simulink model "Energy_Storage_Project_2023a"  (R2023a)
settings: Solver=ode15s  StartTime=0.0  StopTime=1407  FixedStep=0.02  MaxStep=0.1  RelTol=1e-3
undefined symbols (not defined in the file or in its folder): C1, C2, par_balancing_type, R0, R1, R2, R_balance, SoC, V0, V1, V2, V3, V_ocv
libraries: fl_lib x44, nesl_utility x40, ee_lib x8
settings Model: NumberOfSteps=100  Creator=venka  LastModifiedBy=venka
settings RTWCC: GPUComputeCapability=5.0
settings ConfigComp: CovBoundaryAbsTol=1.0e-5

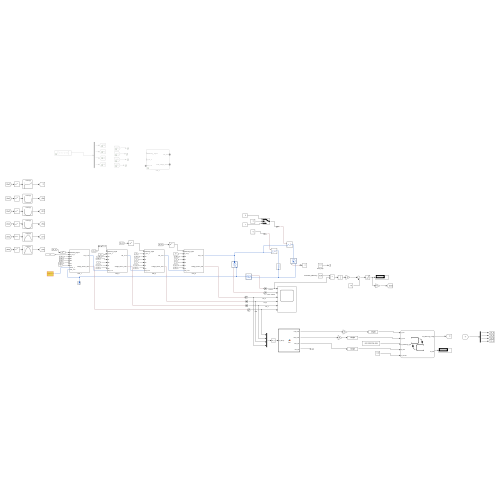
[thumbnail: Simulink's stored preview of the top-level diagram]
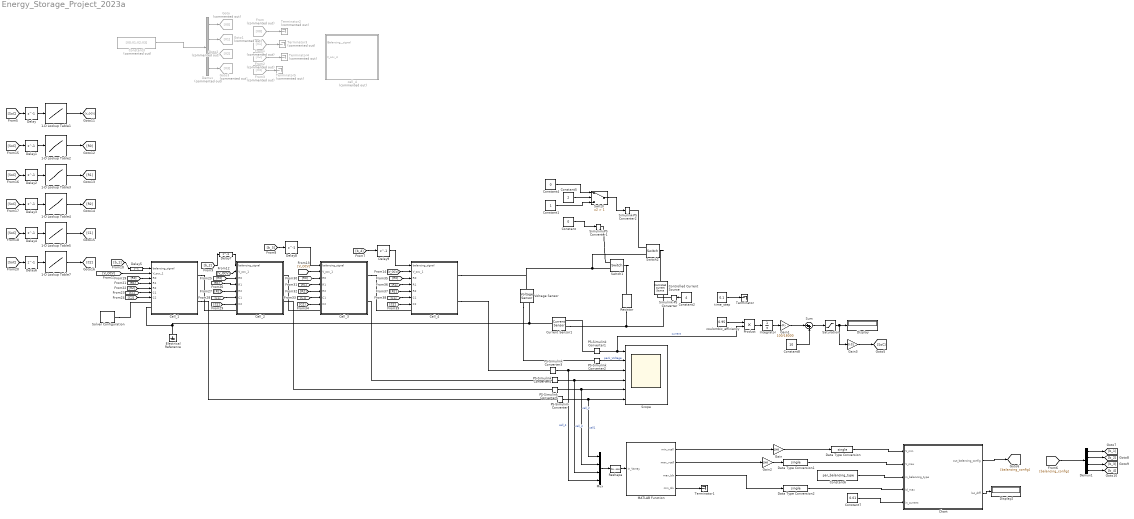
== system Energy_Storage_Project_2023a ==
  1-D Lookup Table1 : Lookup_n-D  NumberOfTableDimensions=1  BreakpointsForDimension1=SoC  Table=V_ocv  InternalRulePriority=Speed  RndMeth=Simplest
  1-D Lookup Table2 : Lookup_n-D  NumberOfTableDimensions=1  BreakpointsForDimension1=SoC  Table=R0  InternalRulePriority=Speed  RndMeth=Simplest
  1-D Lookup Table3 : Lookup_n-D  NumberOfTableDimensions=1  BreakpointsForDimension1=SoC  Table=R1  InternalRulePriority=Speed  RndMeth=Simplest
  1-D Lookup Table4 : Lookup_n-D  NumberOfTableDimensions=1  BreakpointsForDimension1=SoC  Table=R2  InternalRulePriority=Speed  RndMeth=Simplest
  1-D Lookup Table5 : Lookup_n-D  NumberOfTableDimensions=1  BreakpointsForDimension1=SoC  Table=C1  InternalRulePriority=Speed  RndMeth=Simplest
  1-D Lookup Table7 : Lookup_n-D  NumberOfTableDimensions=1  BreakpointsForDimension1=SoC  Table=C2  InternalRulePriority=Speed  RndMeth=Simplest
  Cell_1 : Subsystem
  Cell_2 : Subsystem
  Cell_3 : Subsystem
  Cell_4 : Subsystem
  Chart : Stateflow chart  TreatAsAtomicUnit=on
  Constant : Constant  Value=0
  Constant1 : Constant
  Constant2 : Constant  Value=4
  Constant3 : Constant  Commented=on  Value=[V0;V1;V2;V3]
  Constant4 : Constant  Value=0
  Constant5 : Constant  Value=2
  Constant6 : Constant  Value=par_balancing_type
  Constant7 : Constant  Value=0.01
  Constant8 : Constant  Value=10
  Controlled Current Source : fl_lib/Electrical/Electrical Sources/Controlled Current Source
  Current Sensor1 : fl_lib/Electrical/Electrical Sensors/Current Sensor
  Data Type Conversion : DataTypeConversion  OutDataTypeStr=single  SaturateOnIntegerOverflow=off  RndMeth=Floor
  Data Type Conversion1 : DataTypeConversion  OutDataTypeStr=single  SaturateOnIntegerOverflow=off  RndMeth=Floor
  Data Type Conversion2 : DataTypeConversion  OutDataTypeStr=single  SaturateOnIntegerOverflow=off  RndMeth=Floor
  Delay{,1..9} (10 alike) : Delay  DelayLength=1  InputProcessing=Columns as channels (frame based)
  Demux : Demux  Commented=on
  Demux1 : Demux
  Display : Display
  Display2 : Display
  Electrical Reference : fl_lib/Electrical/Electrical Elements/Electrical Reference
  From : From  Commented=on  GotoTag=V0
  From1 : From  Commented=on  GotoTag=V1
  From2 : From  Commented=on  GotoTag=V2
  From3 : From  Commented=on  GotoTag=V3
  Gain : Gain  Gain=1000
  Gain1 : Gain  Gain=100/18000
  Gain2 : Gain  Gain=1000
  Gain3 : Gain  Gain=0.01
  Goto : Goto  Commented=on  GotoTag=V0
  Goto1 : Goto  Commented=on  GotoTag=V1
  Goto2 : Goto  Commented=on  GotoTag=V2
  Goto3 : Goto  Commented=on  GotoTag=V3
  Integrator : Integrator
  MATLAB Function : MATLAB Function  TreatAsAtomicUnit=on
  Mux : Mux
  PS-Simulink Converter{,1..5} (6 alike) : nesl_utility/PS-Simulink Converter  PhysicalDomain=network_engine_domain  SubClassName=ps_output  LeftPortType=input  RightPortType=output  PseudoPeriodic=off  Frequencies=[]  VectorFormat=inherit  Unit=inherit  AffineConversion=off
  Product : Product
  Reshape : Reshape
  Resistor : fl_lib/Electrical/Electrical Elements/Resistor  R=0.33 Ohm  i_specify=off  i_priority=None  i=0 A  i_nominal_specify=off  i_nominal_value=1  i_nominal_unit=A  v_specify=off  v_priority=None  v=0 V  v_nominal_specify=off  v_nominal_value=1  v_nominal_unit=V
  Saturation : Saturate  UpperLimit=100  LowerLimit=0
  Scope : Scope  NumInputPorts=6
  Simulink-PS Converter : nesl_utility/Simulink-PS Converter  PhysicalDomain=network_engine_domain  SubClassName=ps_input  LeftPortType=input  RightPortType=output  PseudoPeriodic=off  Frequencies=[]  NoiseDistribution=none  NoiseParameters=[]  Unit=1  AffineConversion=off  FilteringAndDerivatives=provide  SimscapeFilterOrder=1  InputFilterTimeConstant=0.001  UdotUserProvided=0
  Simulink-PS Converter1 : nesl_utility/Simulink-PS Converter  PhysicalDomain=network_engine_domain  SubClassName=ps_input  LeftPortType=input  RightPortType=output  PseudoPeriodic=off  Frequencies=[]  NoiseDistribution=none  NoiseParameters=[]  Unit=1  AffineConversion=off  FilteringAndDerivatives=provide  SimscapeFilterOrder=1  InputFilterTimeConstant=0.001  UdotUserProvided=0
  Simulink-PS Converter2 : nesl_utility/Simulink-PS Converter  PhysicalDomain=network_engine_domain  SubClassName=ps_input  LeftPortType=input  RightPortType=output  PseudoPeriodic=off  Frequencies=[]  NoiseDistribution=none  NoiseParameters=[]  Unit=1  AffineConversion=off  FilteringAndDerivatives=provide  SimscapeFilterOrder=1  InputFilterTimeConstant=0.001  UdotUserProvided=0
  Solver Configuration : nesl_utility/Solver Configuration  PhysicalDomain=network_engine_domain  SubClassName=solver  LeftPortType=input  RightPortType=generic  Tones=[]  Harmonics=[]  SimulateNoise=off  Profile=off  UseLocalSampling=off  EnableSwitchedLinearOptims=on  FrequencyDomain=off  UseCCode=off  RelTol=0.001  AbsTol=0.001  MinStep=1e-09  ToWorkspace=off  RevertToSquareIcSolve=off  NumHomotopyIterations=100  PhasorMode=off  PhasorModeNumHarmonics=1  ConsistencySolver=NEWTON_XTOL_AFTER_FTOL  IndexReductionMethod=DerivativeReplacement  DoDC=off  ResidualTolerance=1e-09  ConsistencyTolSource=GLOBAL  ConsistencyAbsTol=0.001  ConsistencyRelTol=0.001  ConsistencyTolFactor=0.001  UseLocalSolver=off  LocalSolverChoice=NE_BACKWARD_EULER_ADVANCER  ResolveIndetEquations=on  FunctionEvalNumThread=1  LocalSolverSampleTime=0.001  DoFixedCost=off  MaxNonlinIter=3  MaxModeIter=2  ComputeImpulses=off  ImpulseIterations=2  LinearAlgebra=auto  LinearAlgebraNumThread=0  EquationFormulation=NE_TIME_EF  DelaysMemoryBudget=1024  AutomaticFiltering=on  FilteringTimeConstant=0.001  PartitionStorageMethod=AS_NEEDED  PartitionMemoryBudget=1024  PartitionMethod=ROBUST  MultibodyUseLocalSolver=off  MultibodyLocalSolverChoice=ODE1  MultibodyLocalSolverSampleTime=0.001
  Sum : Sum  Inputs=|++
  Switch : Switch  Criteria=u2 > Threshold  Threshold=1  SaturateOnIntegerOverflow=off  InputSameDT=off
  Switch1 : fl_lib/Electrical/Electrical Elements/Switch  R_closed=0.01 Ohm  G_open=1e-8 1/Ohm  Threshold=0.5  i_specify=off  i_priority=None  i=0 A  i_nominal_specify=off  i_nominal_value=1  i_nominal_unit=A  v_specify=off  v_priority=None  v=0 V  v_nominal_specify=off  v_nominal_value=1  v_nominal_unit=V
  Switch2 : fl_lib/Electrical/Electrical Elements/Switch  R_closed=0.01 Ohm  G_open=1e-8 1/Ohm  Threshold=0.5  i_specify=off  i_priority=None  i=0 A  i_nominal_specify=off  i_nominal_value=1  i_nominal_unit=A  v_specify=off  v_priority=None  v=0 V  v_nominal_specify=off  v_nominal_value=1  v_nominal_unit=V
  Terminator : Terminator
  Terminator1 : Terminator
  Terminator{2..5} (4 alike) : Terminator  Commented=on
  Voltage Sensor : fl_lib/Electrical/Electrical Sensors/Voltage Sensor
  cell_4 : Subsystem  Commented=on
  coulombic_efficiency : Constant  Value=0.95
  time_step : Constant  Value=0.1
  wires:
  PS-Simulink Converter/1 -> Scope/6, Mux/1  "cell1"
  PS-Simulink Converter1/1 -> Product/2, Scope/1  "current"
  PS-Simulink Converter2/1 -> Scope/2  "pack_Voltage"
  PS-Simulink Converter3/1 -> Mux/4, Scope/3  "cell_4"
  PS-Simulink Converter4/1 -> Mux/3, Scope/4  "cell_3"
  PS-Simulink Converter5/1 -> Scope/5, Mux/2  "cell_2"
  Constant2/1 -> Simulink-PS Converter/1
  Constant/1 -> Simulink-PS Converter1/1
  Constant3/1 -> Demux/1
  Demux/1 -> Goto/1
  Demux/2 -> Goto1/1
  Demux/3 -> Goto2/1
  Demux/4 -> Goto3/1
  time_step/1 -> Terminator/1
  coulombic_efficiency/1 -> Product/1
  Integrator/1 -> Gain1/1
  Product/1 -> Integrator/1
  Sum/1 -> Saturation/1
  Gain1/1 -> Sum/1
  Saturation/1 -> Gain3/1, Display/1
  Constant1/1 -> Switch/3
  Switch/1 -> Simulink-PS Converter2/1
  Constant4/1 -> Switch/1
  MATLAB Function/1(min_vcell) -> Gain/1
  MATLAB Function/2(max_vcell) -> Gain2/1
  Constant6/1 -> Chart/3(in_balancing_type)
  Data Type Conversion/1 -> Chart/1(V_min)
  Data Type Conversion1/1 -> Chart/2(V_max)
  MATLAB Function/3(max_Idx) -> Data Type Conversion2/1
  Data Type Conversion2/1 -> Chart/4(Id_max)
  [balancing_config] -> Demux1/1
  Demux1/1 -> [b_1]
  Demux1/2 -> [b_2]
  Demux1/3 -> [b_3]
  Demux1/4 -> [b_4]
  [b_3] -> Delay8/1
  Chart/1(out_balancing_config) -> [balancing_config]
  Constant5/1 -> Switch/2
  MATLAB Function/4(min_Idx) -> Terminator1/1
  Constant7/1 -> Chart/5(in_current)
  Gain/1 -> Data Type Conversion/1
  Gain2/1 -> Data Type Conversion1/1
  Chart/2(loc_diff) -> Display2/1
  From/1 -> Terminator2/1
  From1/1 -> Terminator3/1
  From2/1 -> Terminator4/1
  From3/1 -> Terminator5/1
  [SoC] -> Delay/1
  Delay/1 -> 1-D Lookup Table1/1
  1-D Lookup Table1/1 -> [V_OCV]
  [V_OCV] -> Cell_1/2(V_ocv_1)
  [V_OCV] -> Cell_2/2(V_ocv_1)
  [V_OCV] -> Cell_3/2(V_ocv_1)
  Constant8/1 -> Sum/2
  1-D Lookup Table2/1 -> [R0]
  [SoC] -> Delay1/1
  Delay1/1 -> 1-D Lookup Table2/1
  1-D Lookup Table3/1 -> [R1]
  [SoC] -> Delay2/1
  Delay2/1 -> 1-D Lookup Table3/1
  1-D Lookup Table4/1 -> [R2]
  [SoC] -> Delay3/1
  Delay3/1 -> 1-D Lookup Table4/1
  1-D Lookup Table5/1 -> [C1]
  [SoC] -> Delay4/1
  Delay4/1 -> 1-D Lookup Table5/1
  [b_4] -> Delay9/1
  [V_OCV] -> Cell_4/2(V_ocv_1)
  Delay6/1 -> 1-D Lookup Table7/1
  1-D Lookup Table7/1 -> [C2]
  [SoC] -> Delay6/1
  [R0] -> Cell_1/3(R0)
  [R1] -> Cell_1/4(R1)
  [R2] -> Cell_1/5(R2)
  [C1] -> Cell_1/6(C1)
  [C2] -> Cell_1/7(C2)
  [R1] -> Cell_2/4(R1)
  [R2] -> Cell_2/5(R2)
  [C2] -> Cell_2/7(C2)
  [C1] -> Cell_2/6(C1)
  [R0] -> Cell_2/3(R0)
  [R1] -> Cell_3/4(R1)
  [R2] -> Cell_3/5(R2)
  [C2] -> Cell_3/7(C2)
  [C1] -> Cell_3/6(C1)
  [R0] -> Cell_3/3(R0)
  [R1] -> Cell_4/4(R1)
  [R2] -> Cell_4/5(R2)
  [C2] -> Cell_4/7(C2)
  [C1] -> Cell_4/6(C1)
  [R0] -> Cell_4/3(R0)
  Mux/1 -> Reshape/1
  Reshape/1 -> MATLAB Function/1(in_Varray)
  [b_1] -> Delay5/1
  Delay5/1 -> Cell_1/1(balancing_signal)
  [b_2] -> Delay7/1
  Delay7/1 -> Cell_2/1(balancing_signal)
  Delay8/1 -> Cell_3/1(balancing_signal)
  Delay9/1 -> Cell_4/1(balancing_signal)
  Gain3/1 -> [SoC]
  connections:
  Switch2/RConn2 -- Cell_4/RConn1 -- Voltage Sensor/LConn1 -- Switch1/RConn2
  Switch1/LConn1 -- Resistor/LConn1
  Solver Configuration/RConn1 -- Cell_1/LConn1
  Cell_1/RConn1 -- Cell_2/LConn1
  Cell_3/LConn1 -- Cell_2/RConn1
  Electrical Reference/LConn1 -- Voltage Sensor/RConn2 -- Current Sensor1/LConn1 -- Cell_1/LConn2
  Cell_1/RConn2 -- PS-Simulink Converter/LConn1
  PS-Simulink Converter5/LConn1 -- Cell_2/RConn2
  PS-Simulink Converter4/LConn1 -- Cell_3/RConn2
  PS-Simulink Converter1/LConn1 -- Current Sensor1/RConn1
  Voltage Sensor/RConn1 -- PS-Simulink Converter2/LConn1
  Switch1/RConn1 -- Simulink-PS Converter1/RConn1
  Resistor/RConn1 -- Current Sensor1/RConn2 -- Controlled Current Source/RConn2
  Switch2/LConn1 -- Controlled Current Source/LConn1
  Switch2/RConn1 -- Simulink-PS Converter2/RConn1
  Simulink-PS Converter/RConn1 -- Controlled Current Source/RConn1
  Cell_3/RConn1 -- Cell_4/LConn1
  Cell_4/RConn2 -- PS-Simulink Converter3/LConn1

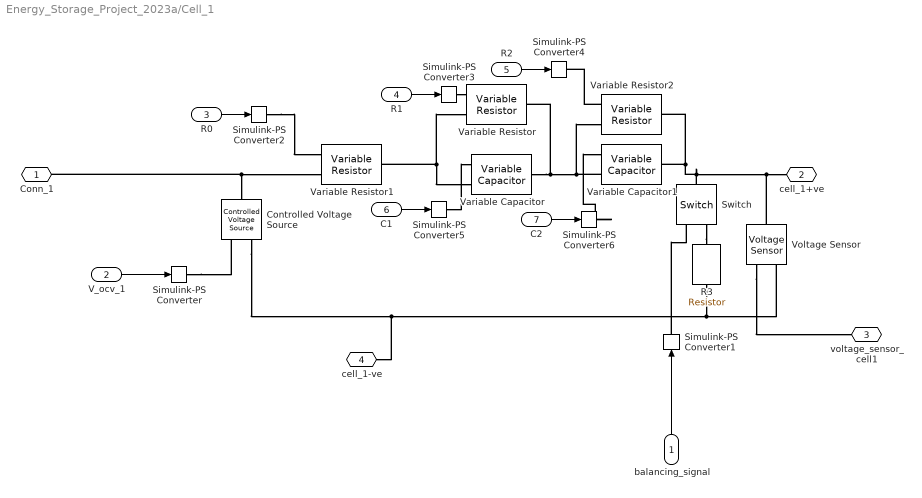
== system Energy_Storage_Project_2023a/Cell_1 ==
  balancing_signal : Inport
  V_ocv_1 : Inport  Port=2
  R0 : Inport  Port=3
  R1 : Inport  Port=4
  R2 : Inport  Port=5
  C1 : Inport  Port=6
  C2 : Inport  Port=7
  Controlled Voltage Source : fl_lib/Electrical/Electrical Sources/Controlled Voltage Source
  R3 : fl_lib/Electrical/Electrical Elements/Resistor  R=R_balance Ohm  i_specify=off  i_priority=None  i=0 A  i_nominal_specify=off  i_nominal_value=1  i_nominal_unit=A  v_specify=off  v_priority=None  v=0 V  v_nominal_specify=off  v_nominal_value=1  v_nominal_unit=V
  Simulink-PS Converter{,1..6} (7 alike) : nesl_utility/Simulink-PS Converter  PhysicalDomain=network_engine_domain  SubClassName=ps_input  LeftPortType=input  RightPortType=output  PseudoPeriodic=off  Frequencies=[]  NoiseDistribution=none  NoiseParameters=[]  Unit=1  AffineConversion=off  FilteringAndDerivatives=provide  SimscapeFilterOrder=1  InputFilterTimeConstant=0.001  UdotUserProvided=0
  Switch : fl_lib/Electrical/Electrical Elements/Switch  R_closed=0.01 Ohm  G_open=1e-8 1/Ohm  Threshold=0.5  i_specify=off  i_priority=None  i=0 A  i_nominal_specify=off  i_nominal_value=1  i_nominal_unit=A  v_specify=off  v_priority=None  v=0 V  v_nominal_specify=off  v_nominal_value=1  v_nominal_unit=V
  Variable Capacitor : ee_lib/Passive/Variable Capacitor  prm=2  Cmin=1e-9 F  r=1e-6 Ohm  v0=0 V  q0=0 C
      settings: InternalSimscapePortConfiguration="{\"Bottom\":[],\"Left\":[{\"id\":\"C\",\"label\":\"C\",\"type\":\"input\"},{\"id\":\"p\",\"label\":\"+\",\"type\":\"foundation.electrical.electrical\"}],\"Right\":[{\"id\":\"n\",\"label\":\"-\",\"type\":\"foundation.electrical.electrical\"}],\"Top\":[]}"
  Variable Capacitor1 : ee_lib/Passive/Variable Capacitor  prm=2  Cmin=1e-9 F  r=1e-6 Ohm  v0=0 V  q0=0 C
      settings: InternalSimscapePortConfiguration="{\"Bottom\":[],\"Left\":[{\"id\":\"C\",\"label\":\"C\",\"type\":\"input\"},{\"id\":\"p\",\"label\":\"+\",\"type\":\"foundation.electrical.electrical\"}],\"Right\":[{\"id\":\"n\",\"label\":\"-\",\"type\":\"foundation.electrical.electrical\"}],\"Top\":[]}"
  Variable Resistor : fl_lib/Electrical/Electrical Elements/Variable Resistor  Rmin=0 Ohm  thermalEnable=false  thermal_mass=1 J/K  i_specify=off  i_priority=None  i=0 A  i_nominal_specify=off  i_nominal_value=1  i_nominal_unit=A  v_specify=off  v_priority=None  v=0 V  v_nominal_specify=off  v_nominal_value=1  v_nominal_unit=V  T_specify=off  T_priority=None  T=300 K  T_nominal_specify=off  T_nominal_value=1  T_nominal_unit=K
  Variable Resistor1 : fl_lib/Electrical/Electrical Elements/Variable Resistor  Rmin=0 Ohm  thermalEnable=false  thermal_mass=1 J/K  i_specify=off  i_priority=None  i=0 A  i_nominal_specify=off  i_nominal_value=1  i_nominal_unit=A  v_specify=off  v_priority=None  v=0 V  v_nominal_specify=off  v_nominal_value=1  v_nominal_unit=V  T_specify=off  T_priority=None  T=300 K  T_nominal_specify=off  T_nominal_value=1  T_nominal_unit=K
  Variable Resistor2 : fl_lib/Electrical/Electrical Elements/Variable Resistor  Rmin=0 Ohm  thermalEnable=false  thermal_mass=1 J/K  i_specify=off  i_priority=None  i=0 A  i_nominal_specify=off  i_nominal_value=1  i_nominal_unit=A  v_specify=off  v_priority=None  v=0 V  v_nominal_specify=off  v_nominal_value=1  v_nominal_unit=V  T_specify=off  T_priority=None  T=300 K  T_nominal_specify=off  T_nominal_value=1  T_nominal_unit=K
  Voltage Sensor : fl_lib/Electrical/Electrical Sensors/Voltage Sensor
  Conn_1 : PMIOPort  Side=Left
  cell_1+ve : PMIOPort  Port=2  Side=Right
  voltage_sensor_cell1 : PMIOPort  Port=3  Side=Right
  cell_1-ve : PMIOPort  Port=4  Side=Left
  wires:
  V_ocv_1/1 -> Simulink-PS Converter/1
  balancing_signal/1 -> Simulink-PS Converter1/1
  R0/1 -> Simulink-PS Converter2/1
  R1/1 -> Simulink-PS Converter3/1
  R2/1 -> Simulink-PS Converter4/1
  C1/1 -> Simulink-PS Converter5/1
  C2/1 -> Simulink-PS Converter6/1
  connections:
  Voltage Sensor/LConn1 -- Variable Capacitor1/RConn1 -- Variable Resistor2/RConn1 -- Switch/LConn1 -- cell_1+ve/RConn1
  Variable Resistor1/RConn1 -- Variable Resistor/LConn2 -- Variable Capacitor/LConn2
  Variable Capacitor/RConn1 -- Variable Resistor/RConn1 -- Variable Capacitor1/LConn2 -- Variable Resistor2/LConn2
  cell_1-ve/RConn1 -- Controlled Voltage Source/RConn2 -- R3/RConn1 -- Voltage Sensor/RConn2
  Voltage Sensor/RConn1 -- voltage_sensor_cell1/RConn1
  Conn_1/RConn1 -- Variable Resistor1/LConn2 -- Controlled Voltage Source/LConn1
  Simulink-PS Converter/RConn1 -- Controlled Voltage Source/RConn1
  Switch/RConn2 -- R3/LConn1
  Simulink-PS Converter1/RConn1 -- Switch/RConn1
  Simulink-PS Converter2/RConn1 -- Variable Resistor1/LConn1
  Simulink-PS Converter3/RConn1 -- Variable Resistor/LConn1
  Variable Resistor2/LConn1 -- Simulink-PS Converter4/RConn1
  Simulink-PS Converter5/RConn1 -- Variable Capacitor/LConn1
  Simulink-PS Converter6/RConn1 -- Variable Capacitor1/LConn1

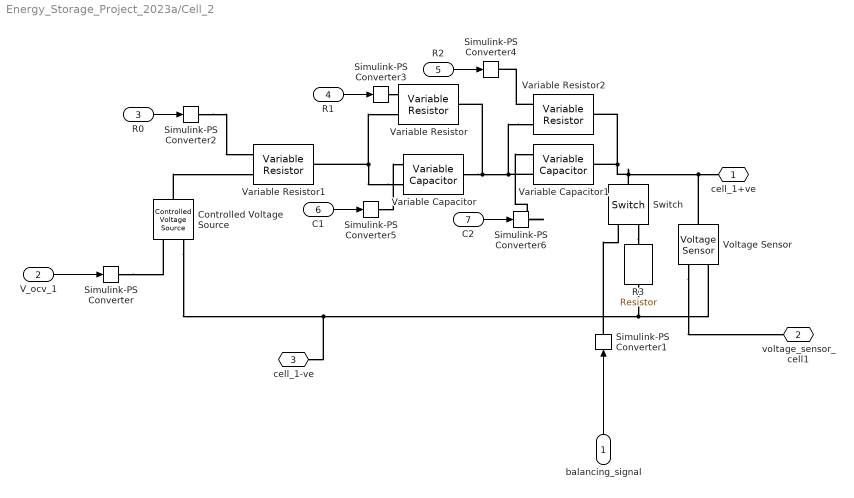
== system Energy_Storage_Project_2023a/Cell_2 ==
  balancing_signal : Inport
  V_ocv_1 : Inport  Port=2
  R0 : Inport  Port=3
  R1 : Inport  Port=4
  R2 : Inport  Port=5
  C1 : Inport  Port=6
  C2 : Inport  Port=7
  Controlled Voltage Source : fl_lib/Electrical/Electrical Sources/Controlled Voltage Source
  R3 : fl_lib/Electrical/Electrical Elements/Resistor  R=R_balance Ohm  i_specify=off  i_priority=None  i=0 A  i_nominal_specify=off  i_nominal_value=1  i_nominal_unit=A  v_specify=off  v_priority=None  v=0 V  v_nominal_specify=off  v_nominal_value=1  v_nominal_unit=V
  Simulink-PS Converter{,1..6} (7 alike) : nesl_utility/Simulink-PS Converter  PhysicalDomain=network_engine_domain  SubClassName=ps_input  LeftPortType=input  RightPortType=output  PseudoPeriodic=off  Frequencies=[]  NoiseDistribution=none  NoiseParameters=[]  Unit=1  AffineConversion=off  FilteringAndDerivatives=provide  SimscapeFilterOrder=1  InputFilterTimeConstant=0.001  UdotUserProvided=0
  Switch : fl_lib/Electrical/Electrical Elements/Switch  R_closed=0.01 Ohm  G_open=1e-8 1/Ohm  Threshold=0.5  i_specify=off  i_priority=None  i=0 A  i_nominal_specify=off  i_nominal_value=1  i_nominal_unit=A  v_specify=off  v_priority=None  v=0 V  v_nominal_specify=off  v_nominal_value=1  v_nominal_unit=V
  Variable Capacitor : ee_lib/Passive/Variable Capacitor  prm=2  Cmin=1e-9 F  r=1e-6 Ohm  v0=0 V  q0=0 C
      settings: InternalSimscapePortConfiguration="{\"Bottom\":[],\"Left\":[{\"id\":\"C\",\"label\":\"C\",\"type\":\"input\"},{\"id\":\"p\",\"label\":\"+\",\"type\":\"foundation.electrical.electrical\"}],\"Right\":[{\"id\":\"n\",\"label\":\"-\",\"type\":\"foundation.electrical.electrical\"}],\"Top\":[]}"
  Variable Capacitor1 : ee_lib/Passive/Variable Capacitor  prm=2  Cmin=1e-9 F  r=1e-6 Ohm  v0=0 V  q0=0 C
      settings: InternalSimscapePortConfiguration="{\"Bottom\":[],\"Left\":[{\"id\":\"C\",\"label\":\"C\",\"type\":\"input\"},{\"id\":\"p\",\"label\":\"+\",\"type\":\"foundation.electrical.electrical\"}],\"Right\":[{\"id\":\"n\",\"label\":\"-\",\"type\":\"foundation.electrical.electrical\"}],\"Top\":[]}"
  Variable Resistor : fl_lib/Electrical/Electrical Elements/Variable Resistor  Rmin=0 Ohm  thermalEnable=false  thermal_mass=1 J/K  i_specify=off  i_priority=None  i=0 A  i_nominal_specify=off  i_nominal_value=1  i_nominal_unit=A  v_specify=off  v_priority=None  v=0 V  v_nominal_specify=off  v_nominal_value=1  v_nominal_unit=V  T_specify=off  T_priority=None  T=300 K  T_nominal_specify=off  T_nominal_value=1  T_nominal_unit=K
  Variable Resistor1 : fl_lib/Electrical/Electrical Elements/Variable Resistor  Rmin=0 Ohm  thermalEnable=false  thermal_mass=1 J/K  i_specify=off  i_priority=None  i=0 A  i_nominal_specify=off  i_nominal_value=1  i_nominal_unit=A  v_specify=off  v_priority=None  v=0 V  v_nominal_specify=off  v_nominal_value=1  v_nominal_unit=V  T_specify=off  T_priority=None  T=300 K  T_nominal_specify=off  T_nominal_value=1  T_nominal_unit=K
  Variable Resistor2 : fl_lib/Electrical/Electrical Elements/Variable Resistor  Rmin=0 Ohm  thermalEnable=false  thermal_mass=1 J/K  i_specify=off  i_priority=None  i=0 A  i_nominal_specify=off  i_nominal_value=1  i_nominal_unit=A  v_specify=off  v_priority=None  v=0 V  v_nominal_specify=off  v_nominal_value=1  v_nominal_unit=V  T_specify=off  T_priority=None  T=300 K  T_nominal_specify=off  T_nominal_value=1  T_nominal_unit=K
  Voltage Sensor : fl_lib/Electrical/Electrical Sensors/Voltage Sensor
  cell_1+ve : PMIOPort  Side=Right
  voltage_sensor_cell1 : PMIOPort  Port=2  Side=Right
  cell_1-ve : PMIOPort  Port=3  Side=Left
  wires:
  V_ocv_1/1 -> Simulink-PS Converter/1
  balancing_signal/1 -> Simulink-PS Converter1/1
  R0/1 -> Simulink-PS Converter2/1
  R1/1 -> Simulink-PS Converter3/1
  R2/1 -> Simulink-PS Converter4/1
  C1/1 -> Simulink-PS Converter5/1
  C2/1 -> Simulink-PS Converter6/1
  connections:
  Voltage Sensor/LConn1 -- cell_1+ve/RConn1 -- Switch/LConn1 -- Variable Resistor2/RConn1 -- Variable Capacitor1/RConn1
  Variable Capacitor/LConn2 -- Variable Resistor1/RConn1 -- Variable Resistor/LConn2
  Variable Resistor2/LConn2 -- Variable Capacitor/RConn1 -- Variable Resistor/RConn1 -- Variable Capacitor1/LConn2
  cell_1-ve/RConn1 -- Controlled Voltage Source/RConn2 -- R3/RConn1 -- Voltage Sensor/RConn2
  Voltage Sensor/RConn1 -- voltage_sensor_cell1/RConn1
  Controlled Voltage Source/LConn1 -- Variable Resistor1/LConn2
  Simulink-PS Converter/RConn1 -- Controlled Voltage Source/RConn1
  Switch/RConn2 -- R3/LConn1
  Simulink-PS Converter1/RConn1 -- Switch/RConn1
  Simulink-PS Converter2/RConn1 -- Variable Resistor1/LConn1
  Simulink-PS Converter3/RConn1 -- Variable Resistor/LConn1
  Variable Resistor2/LConn1 -- Simulink-PS Converter4/RConn1
  Simulink-PS Converter5/RConn1 -- Variable Capacitor/LConn1
  Simulink-PS Converter6/RConn1 -- Variable Capacitor1/LConn1

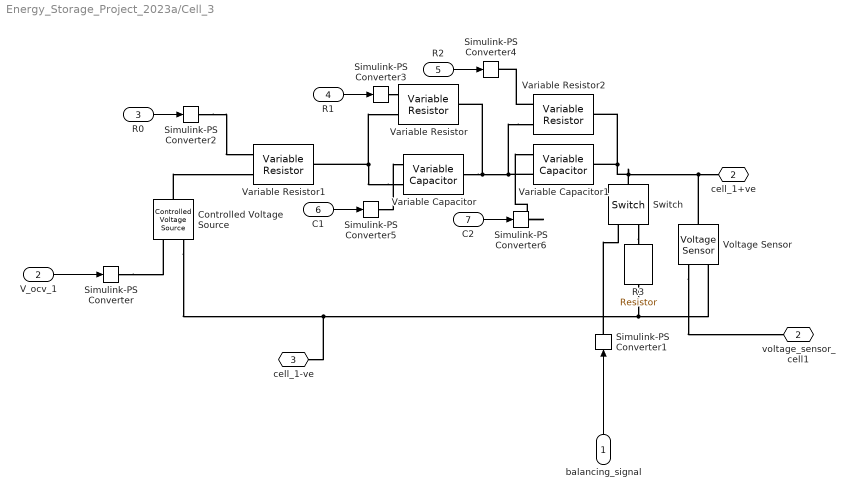
== system Energy_Storage_Project_2023a/Cell_3 ==
  balancing_signal : Inport
  V_ocv_1 : Inport  Port=2
  R0 : Inport  Port=3
  R1 : Inport  Port=4
  R2 : Inport  Port=5
  C1 : Inport  Port=6
  C2 : Inport  Port=7
  Controlled Voltage Source : fl_lib/Electrical/Electrical Sources/Controlled Voltage Source
  R3 : fl_lib/Electrical/Electrical Elements/Resistor  R=R_balance Ohm  i_specify=off  i_priority=None  i=0 A  i_nominal_specify=off  i_nominal_value=1  i_nominal_unit=A  v_specify=off  v_priority=None  v=0 V  v_nominal_specify=off  v_nominal_value=1  v_nominal_unit=V
  Simulink-PS Converter{,1..6} (7 alike) : nesl_utility/Simulink-PS Converter  PhysicalDomain=network_engine_domain  SubClassName=ps_input  LeftPortType=input  RightPortType=output  PseudoPeriodic=off  Frequencies=[]  NoiseDistribution=none  NoiseParameters=[]  Unit=1  AffineConversion=off  FilteringAndDerivatives=provide  SimscapeFilterOrder=1  InputFilterTimeConstant=0.001  UdotUserProvided=0
  Switch : fl_lib/Electrical/Electrical Elements/Switch  R_closed=0.01 Ohm  G_open=1e-8 1/Ohm  Threshold=0.5  i_specify=off  i_priority=None  i=0 A  i_nominal_specify=off  i_nominal_value=1  i_nominal_unit=A  v_specify=off  v_priority=None  v=0 V  v_nominal_specify=off  v_nominal_value=1  v_nominal_unit=V
  Variable Capacitor : ee_lib/Passive/Variable Capacitor  prm=2  Cmin=1e-9 F  r=1e-6 Ohm  v0=0 V  q0=0 C
      settings: InternalSimscapePortConfiguration="{\"Bottom\":[],\"Left\":[{\"id\":\"C\",\"label\":\"C\",\"type\":\"input\"},{\"id\":\"p\",\"label\":\"+\",\"type\":\"foundation.electrical.electrical\"}],\"Right\":[{\"id\":\"n\",\"label\":\"-\",\"type\":\"foundation.electrical.electrical\"}],\"Top\":[]}"
  Variable Capacitor1 : ee_lib/Passive/Variable Capacitor  prm=2  Cmin=1e-9 F  r=1e-6 Ohm  v0=0 V  q0=0 C
      settings: InternalSimscapePortConfiguration="{\"Bottom\":[],\"Left\":[{\"id\":\"C\",\"label\":\"C\",\"type\":\"input\"},{\"id\":\"p\",\"label\":\"+\",\"type\":\"foundation.electrical.electrical\"}],\"Right\":[{\"id\":\"n\",\"label\":\"-\",\"type\":\"foundation.electrical.electrical\"}],\"Top\":[]}"
  Variable Resistor : fl_lib/Electrical/Electrical Elements/Variable Resistor  Rmin=0 Ohm  thermalEnable=false  thermal_mass=1 J/K  i_specify=off  i_priority=None  i=0 A  i_nominal_specify=off  i_nominal_value=1  i_nominal_unit=A  v_specify=off  v_priority=None  v=0 V  v_nominal_specify=off  v_nominal_value=1  v_nominal_unit=V  T_specify=off  T_priority=None  T=300 K  T_nominal_specify=off  T_nominal_value=1  T_nominal_unit=K
  Variable Resistor1 : fl_lib/Electrical/Electrical Elements/Variable Resistor  Rmin=0 Ohm  thermalEnable=false  thermal_mass=1 J/K  i_specify=off  i_priority=None  i=0 A  i_nominal_specify=off  i_nominal_value=1  i_nominal_unit=A  v_specify=off  v_priority=None  v=0 V  v_nominal_specify=off  v_nominal_value=1  v_nominal_unit=V  T_specify=off  T_priority=None  T=300 K  T_nominal_specify=off  T_nominal_value=1  T_nominal_unit=K
  Variable Resistor2 : fl_lib/Electrical/Electrical Elements/Variable Resistor  Rmin=0 Ohm  thermalEnable=false  thermal_mass=1 J/K  i_specify=off  i_priority=None  i=0 A  i_nominal_specify=off  i_nominal_value=1  i_nominal_unit=A  v_specify=off  v_priority=None  v=0 V  v_nominal_specify=off  v_nominal_value=1  v_nominal_unit=V  T_specify=off  T_priority=None  T=300 K  T_nominal_specify=off  T_nominal_value=1  T_nominal_unit=K
  Voltage Sensor : fl_lib/Electrical/Electrical Sensors/Voltage Sensor
  cell_1-ve : PMIOPort  Port=3  Side=Left
  cell_1+ve : PMIOPort  Port=2  Side=Right
  voltage_sensor_cell1 : PMIOPort  Port=2  Side=Right
  wires:
  V_ocv_1/1 -> Simulink-PS Converter/1
  balancing_signal/1 -> Simulink-PS Converter1/1
  R0/1 -> Simulink-PS Converter2/1
  R1/1 -> Simulink-PS Converter3/1
  R2/1 -> Simulink-PS Converter4/1
  C1/1 -> Simulink-PS Converter5/1
  C2/1 -> Simulink-PS Converter6/1
  connections:
  Voltage Sensor/LConn1 -- cell_1+ve/RConn1 -- Switch/LConn1 -- Variable Resistor2/RConn1 -- Variable Capacitor1/RConn1
  Variable Capacitor/LConn2 -- Variable Resistor1/RConn1 -- Variable Resistor/LConn2
  Variable Resistor2/LConn2 -- Variable Capacitor/RConn1 -- Variable Resistor/RConn1 -- Variable Capacitor1/LConn2
  cell_1-ve/RConn1 -- Controlled Voltage Source/RConn2 -- R3/RConn1 -- Voltage Sensor/RConn2
  Voltage Sensor/RConn1 -- voltage_sensor_cell1/RConn1
  Controlled Voltage Source/LConn1 -- Variable Resistor1/LConn2
  Simulink-PS Converter/RConn1 -- Controlled Voltage Source/RConn1
  Switch/RConn2 -- R3/LConn1
  Simulink-PS Converter1/RConn1 -- Switch/RConn1
  Simulink-PS Converter2/RConn1 -- Variable Resistor1/LConn1
  Simulink-PS Converter3/RConn1 -- Variable Resistor/LConn1
  Variable Resistor2/LConn1 -- Simulink-PS Converter4/RConn1
  Simulink-PS Converter5/RConn1 -- Variable Capacitor/LConn1
  Simulink-PS Converter6/RConn1 -- Variable Capacitor1/LConn1

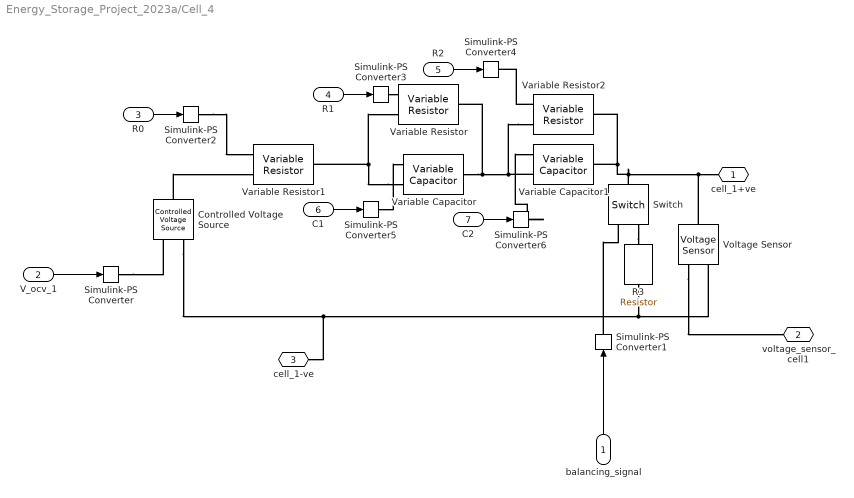
== system Energy_Storage_Project_2023a/Cell_4 ==
  balancing_signal : Inport
  V_ocv_1 : Inport  Port=2
  R0 : Inport  Port=3
  R1 : Inport  Port=4
  R2 : Inport  Port=5
  C1 : Inport  Port=6
  C2 : Inport  Port=7
  Controlled Voltage Source : fl_lib/Electrical/Electrical Sources/Controlled Voltage Source
  R3 : fl_lib/Electrical/Electrical Elements/Resistor  R=R_balance Ohm  i_specify=off  i_priority=None  i=0 A  i_nominal_specify=off  i_nominal_value=1  i_nominal_unit=A  v_specify=off  v_priority=None  v=0 V  v_nominal_specify=off  v_nominal_value=1  v_nominal_unit=V
  Simulink-PS Converter{,1..6} (7 alike) : nesl_utility/Simulink-PS Converter  PhysicalDomain=network_engine_domain  SubClassName=ps_input  LeftPortType=input  RightPortType=output  PseudoPeriodic=off  Frequencies=[]  NoiseDistribution=none  NoiseParameters=[]  Unit=1  AffineConversion=off  FilteringAndDerivatives=provide  SimscapeFilterOrder=1  InputFilterTimeConstant=0.001  UdotUserProvided=0
  Switch : fl_lib/Electrical/Electrical Elements/Switch  R_closed=0.01 Ohm  G_open=1e-8 1/Ohm  Threshold=0.5  i_specify=off  i_priority=None  i=0 A  i_nominal_specify=off  i_nominal_value=1  i_nominal_unit=A  v_specify=off  v_priority=None  v=0 V  v_nominal_specify=off  v_nominal_value=1  v_nominal_unit=V
  Variable Capacitor : ee_lib/Passive/Variable Capacitor  prm=2  Cmin=1e-9 F  r=1e-6 Ohm  v0=0 V  q0=0 C
      settings: InternalSimscapePortConfiguration="{\"Bottom\":[],\"Left\":[{\"id\":\"C\",\"label\":\"C\",\"type\":\"input\"},{\"id\":\"p\",\"label\":\"+\",\"type\":\"foundation.electrical.electrical\"}],\"Right\":[{\"id\":\"n\",\"label\":\"-\",\"type\":\"foundation.electrical.electrical\"}],\"Top\":[]}"
  Variable Capacitor1 : ee_lib/Passive/Variable Capacitor  prm=2  Cmin=1e-9 F  r=1e-6 Ohm  v0=0 V  q0=0 C
      settings: InternalSimscapePortConfiguration="{\"Bottom\":[],\"Left\":[{\"id\":\"C\",\"label\":\"C\",\"type\":\"input\"},{\"id\":\"p\",\"label\":\"+\",\"type\":\"foundation.electrical.electrical\"}],\"Right\":[{\"id\":\"n\",\"label\":\"-\",\"type\":\"foundation.electrical.electrical\"}],\"Top\":[]}"
  Variable Resistor : fl_lib/Electrical/Electrical Elements/Variable Resistor  Rmin=0 Ohm  thermalEnable=false  thermal_mass=1 J/K  i_specify=off  i_priority=None  i=0 A  i_nominal_specify=off  i_nominal_value=1  i_nominal_unit=A  v_specify=off  v_priority=None  v=0 V  v_nominal_specify=off  v_nominal_value=1  v_nominal_unit=V  T_specify=off  T_priority=None  T=300 K  T_nominal_specify=off  T_nominal_value=1  T_nominal_unit=K
  Variable Resistor1 : fl_lib/Electrical/Electrical Elements/Variable Resistor  Rmin=0 Ohm  thermalEnable=false  thermal_mass=1 J/K  i_specify=off  i_priority=None  i=0 A  i_nominal_specify=off  i_nominal_value=1  i_nominal_unit=A  v_specify=off  v_priority=None  v=0 V  v_nominal_specify=off  v_nominal_value=1  v_nominal_unit=V  T_specify=off  T_priority=None  T=300 K  T_nominal_specify=off  T_nominal_value=1  T_nominal_unit=K
  Variable Resistor2 : fl_lib/Electrical/Electrical Elements/Variable Resistor  Rmin=0 Ohm  thermalEnable=false  thermal_mass=1 J/K  i_specify=off  i_priority=None  i=0 A  i_nominal_specify=off  i_nominal_value=1  i_nominal_unit=A  v_specify=off  v_priority=None  v=0 V  v_nominal_specify=off  v_nominal_value=1  v_nominal_unit=V  T_specify=off  T_priority=None  T=300 K  T_nominal_specify=off  T_nominal_value=1  T_nominal_unit=K
  Voltage Sensor : fl_lib/Electrical/Electrical Sensors/Voltage Sensor
  cell_1+ve : PMIOPort  Side=Right
  voltage_sensor_cell1 : PMIOPort  Port=2  Side=Right
  cell_1-ve : PMIOPort  Port=3  Side=Left
  wires:
  V_ocv_1/1 -> Simulink-PS Converter/1
  balancing_signal/1 -> Simulink-PS Converter1/1
  R0/1 -> Simulink-PS Converter2/1
  R1/1 -> Simulink-PS Converter3/1
  R2/1 -> Simulink-PS Converter4/1
  C1/1 -> Simulink-PS Converter5/1
  C2/1 -> Simulink-PS Converter6/1
  connections:
  Voltage Sensor/LConn1 -- cell_1+ve/RConn1 -- Switch/LConn1 -- Variable Resistor2/RConn1 -- Variable Capacitor1/RConn1
  Variable Capacitor/LConn2 -- Variable Resistor1/RConn1 -- Variable Resistor/LConn2
  Variable Resistor2/LConn2 -- Variable Capacitor/RConn1 -- Variable Resistor/RConn1 -- Variable Capacitor1/LConn2
  cell_1-ve/RConn1 -- Controlled Voltage Source/RConn2 -- R3/RConn1 -- Voltage Sensor/RConn2
  Voltage Sensor/RConn1 -- voltage_sensor_cell1/RConn1
  Controlled Voltage Source/LConn1 -- Variable Resistor1/LConn2
  Simulink-PS Converter/RConn1 -- Controlled Voltage Source/RConn1
  Switch/RConn2 -- R3/LConn1
  Simulink-PS Converter1/RConn1 -- Switch/RConn1
  Simulink-PS Converter2/RConn1 -- Variable Resistor1/LConn1
  Simulink-PS Converter3/RConn1 -- Variable Resistor/LConn1
  Variable Resistor2/LConn1 -- Simulink-PS Converter4/RConn1
  Simulink-PS Converter5/RConn1 -- Variable Capacitor/LConn1
  Simulink-PS Converter6/RConn1 -- Variable Capacitor1/LConn1

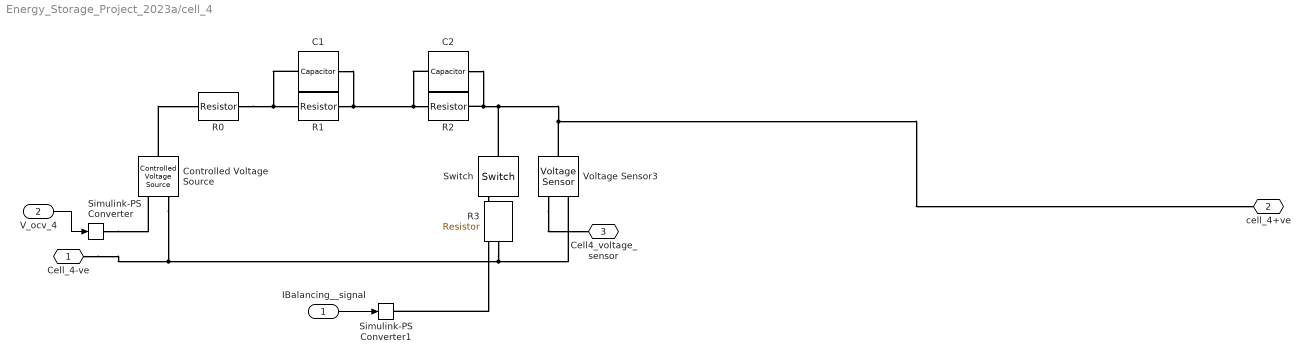
== system Energy_Storage_Project_2023a/cell_4 ==
  IBalancing__signal : Inport
  V_ocv_4 : Inport  Port=2
  C1 : fl_lib/Electrical/Electrical Elements/Capacitor  c=C1 F  r=0 Ohm  g=0 1/Ohm  i_specify=off  i_priority=None  i=0 A  i_nominal_specify=off  i_nominal_value=1  i_nominal_unit=A  v_specify=off  v_priority=None  v=0 V  v_nominal_specify=off  v_nominal_value=1  v_nominal_unit=V  vc_specify=on  vc_priority=High  vc=0 V  vc_nominal_specify=off  vc_nominal_value=1  vc_nominal_unit=V
  C2 : fl_lib/Electrical/Electrical Elements/Capacitor  c=C2 F  r=0 Ohm  g=0 1/Ohm  i_specify=off  i_priority=None  i=0 A  i_nominal_specify=off  i_nominal_value=1  i_nominal_unit=A  v_specify=off  v_priority=None  v=0 V  v_nominal_specify=off  v_nominal_value=1  v_nominal_unit=V  vc_specify=on  vc_priority=High  vc=0 V  vc_nominal_specify=off  vc_nominal_value=1  vc_nominal_unit=V
  Controlled Voltage Source : fl_lib/Electrical/Electrical Sources/Controlled Voltage Source
  R0 : fl_lib/Electrical/Electrical Elements/Resistor  R=R0 Ohm  i_specify=off  i_priority=None  i=0 A  i_nominal_specify=off  i_nominal_value=1  i_nominal_unit=A  v_specify=off  v_priority=None  v=0 V  v_nominal_specify=off  v_nominal_value=1  v_nominal_unit=V
  R1 : fl_lib/Electrical/Electrical Elements/Resistor  R=R1 Ohm  i_specify=off  i_priority=None  i=0 A  i_nominal_specify=off  i_nominal_value=1  i_nominal_unit=A  v_specify=off  v_priority=None  v=0 V  v_nominal_specify=off  v_nominal_value=1  v_nominal_unit=V
  R2 : fl_lib/Electrical/Electrical Elements/Resistor  R=R2 Ohm  i_specify=off  i_priority=None  i=0 A  i_nominal_specify=off  i_nominal_value=1  i_nominal_unit=A  v_specify=off  v_priority=None  v=0 V  v_nominal_specify=off  v_nominal_value=1  v_nominal_unit=V
  R3 : fl_lib/Electrical/Electrical Elements/Resistor  R=R_balance Ohm  i_specify=off  i_priority=None  i=0 A  i_nominal_specify=off  i_nominal_value=1  i_nominal_unit=A  v_specify=off  v_priority=None  v=0 V  v_nominal_specify=off  v_nominal_value=1  v_nominal_unit=V
  Simulink-PS Converter : nesl_utility/Simulink-PS Converter  PhysicalDomain=network_engine_domain  SubClassName=ps_input  LeftPortType=input  RightPortType=output  PseudoPeriodic=off  Frequencies=[]  NoiseDistribution=none  NoiseParameters=[]  Unit=1  AffineConversion=off  FilteringAndDerivatives=provide  SimscapeFilterOrder=1  InputFilterTimeConstant=0.001  UdotUserProvided=0
  Simulink-PS Converter1 : nesl_utility/Simulink-PS Converter  PhysicalDomain=network_engine_domain  SubClassName=ps_input  LeftPortType=input  RightPortType=output  PseudoPeriodic=off  Frequencies=[]  NoiseDistribution=none  NoiseParameters=[]  Unit=1  AffineConversion=off  FilteringAndDerivatives=provide  SimscapeFilterOrder=1  InputFilterTimeConstant=0.001  UdotUserProvided=0
  Switch : fl_lib/Electrical/Electrical Elements/Switch  R_closed=0.01 Ohm  G_open=1e-8 1/Ohm  Threshold=0.5  i_specify=off  i_priority=None  i=0 A  i_nominal_specify=off  i_nominal_value=1  i_nominal_unit=A  v_specify=off  v_priority=None  v=0 V  v_nominal_specify=off  v_nominal_value=1  v_nominal_unit=V
  Voltage Sensor3 : fl_lib/Electrical/Electrical Sensors/Voltage Sensor
  Cell_4-ve : PMIOPort  Side=Left
  cell_4+ve : PMIOPort  Port=2  Side=Right
  Cell4_voltage_sensor : PMIOPort  Port=3  Side=Right
  wires:
  V_ocv_4/1 -> Simulink-PS Converter/1
  IBalancing__signal/1 -> Simulink-PS Converter1/1
  connections:
  R2/RConn1 -- Voltage Sensor3/LConn1 -- cell_4+ve/RConn1 -- Switch/LConn1 -- C2/RConn1
  Cell_4-ve/RConn1 -- Controlled Voltage Source/RConn2 -- R3/RConn1 -- Voltage Sensor3/RConn2
  Voltage Sensor3/RConn1 -- Cell4_voltage_sensor/RConn1
  R1/RConn1 -- C1/RConn1 -- C2/LConn1 -- R2/LConn1
  Controlled Voltage Source/LConn1 -- R0/LConn1
  R0/RConn1 -- C1/LConn1 -- R1/LConn1
  Simulink-PS Converter/RConn1 -- Controlled Voltage Source/RConn1
  Switch/RConn1 -- Simulink-PS Converter1/RConn1

== matlab function Energy_Storage_Project_2023a/MATLAB Function ==
  data: in_Varray input; min_vcell output; max_vcell output; max_Idx output; min_Idx output
function [min_vcell,max_vcell,max_Idx,min_Idx] = fcn(in_Varray)
[min_vcell,min_Idx] = min(in_Varray);
[max_vcell,max_Idx] = max(in_Varray);
end

== stateflow chart Energy_Storage_Project_2023a/Chart ==
  state Passive
    en,du:
    loc_diff=V_max-V_min;
    if V_max-V_min >=50
    for i=1:length(out_balancing_config)
    if i==Id_max
    out_balancing_config(i)=1;
    else
    out_balancing_config(i)=0;
    end
    end
    end
  state init
    en,du:
    out_balancing_config=zeros(1,4);
  state Active
  (default) -> init
  init -> Passive [order 1] : [in_balancing_type==1 &&...
      | in_current <=0.5&&in_current >-0.2]
  Passive -> init : [(V_max-V_min <50)]
  Active -> init : [(V_max-V_min <=500)]
  init -> Active [order 2] : [in_balancing_type==2 && (V_max-V_min >=50)]
  data: V_min input; V_max input; in_balancing_type input; out_balancing_config output; Id_max input; in_current input; i local; loc_diff output
